simulink model "Fuzzy_Regulator"  (Simulink 7.1)
settings: Solver=ode3  StartTime=0.0  StopTime=30  FixedStep=0.01  RelTol=1e-3
libraries: fuzblock x2, simulink_extras x1, simulink x1
settings Model: Creator=Michal  LastModifiedBy=Michal

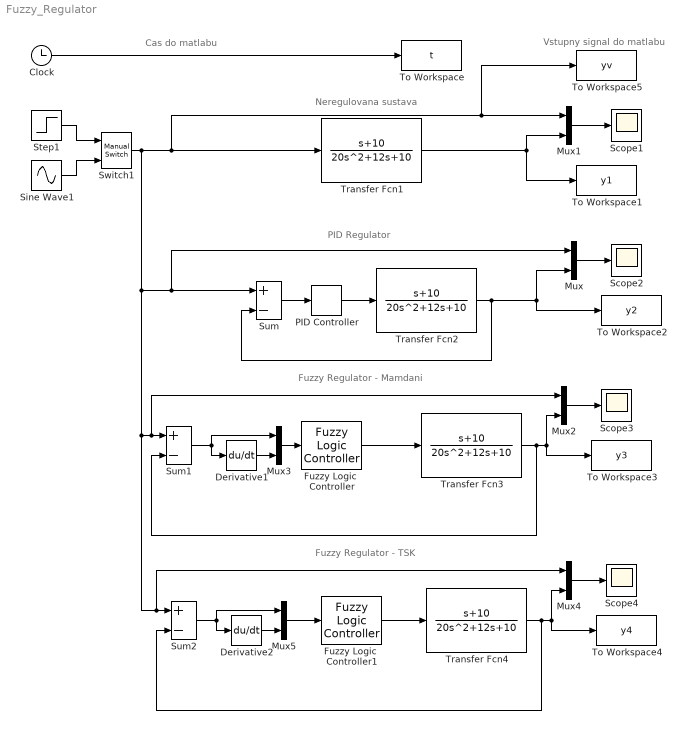
== system Fuzzy_Regulator ==
  note: Cas do matlabu
  note: Neregulovana sustava
  note: PID Regulator
  note: Fuzzy Regulator - Mamdani
  note: Fuzzy Regulator - TSK
  note: Vstupny signal do matlabu
  Clock : Clock
      settings: Decimation=10
  Derivative1 : Derivative
  Derivative2 : Derivative
  Fuzzy Logic  Controller : fuzblock/Fuzzy Logic  Controller  SystemSampleTime=-1  fis='FR_Mamdani.fis'
  Fuzzy Logic  Controller1 : fuzblock/Fuzzy Logic  Controller  SystemSampleTime=-1  fis='FR_TSK.fis'
  Mux{,1..5} (6 alike) : Mux  Inputs=2
  PID Controller : simulink_extras/Additional Linear/PID Controller  SystemSampleTime=-1  P=40  I=2.75  D=20
  Scope{1..4} (4 alike) : Scope
      Scope1 settings: YMin=-4.5e+287  YMax=4.5e+287
      Scope2 settings: YMin=0
      Scope3 settings: YMin=0  SaveName=ScopeData2
      Scope4 settings: TimeRange=20  YMin=-10  YMax=40  SaveName=ScopeData3
  Sine Wave1 : Sin  Bias=10  SampleTime=0
  Step1 : Step  Time=0  After=10  SampleTime=0
  Sum : Sum  Inputs=+|-  OutDataType=sfix(16)  OutScaling=2^0
  Sum1 : Sum  Inputs=+|-  OutDataType=sfix(16)  OutScaling=2^0
  Sum2 : Sum  Inputs=+|-  OutDataType=sfix(16)  OutScaling=2^0
  Switch1 : simulink/Signal Routing/Manual Switch  SystemSampleTime=-1  sw=1  action=0  varsize=off
  To Workspace : ToWorkspace  VariableName=t  SampleTime=-1  SaveFormat=Array
  To Workspace1 : ToWorkspace  VariableName=y1  SampleTime=-1  SaveFormat=Array
  To Workspace2 : ToWorkspace  VariableName=y2  SampleTime=-1  SaveFormat=Array
  To Workspace3 : ToWorkspace  VariableName=y3  SampleTime=-1  SaveFormat=Array
  To Workspace4 : ToWorkspace  VariableName=y4  SampleTime=-1  SaveFormat=Array
  To Workspace5 : ToWorkspace  VariableName=yv  SampleTime=-1  SaveFormat=Array
  Transfer Fcn{1..4} (4 alike) : TransferFcn  Numerator=[1 10]  Denominator=[20 12 10]
  wires:
  Transfer Fcn2/1 -> Sum/2, Mux/2, To Workspace2/1
  PID Controller/1 -> Transfer Fcn2/1
  Sum/1 -> PID Controller/1
  Mux/1 -> Scope2/1
  Mux1/1 -> Scope1/1
  Transfer Fcn1/1 -> Mux1/2, To Workspace1/1
  Transfer Fcn3/1 -> Sum1/2, Mux2/2, To Workspace3/1
  Mux2/1 -> Scope3/1
  Fuzzy Logic  Controller/1 -> Transfer Fcn3/1
  Derivative1/1 -> Mux3/2
  Clock/1 -> To Workspace/1
  Sine Wave1/1 -> Switch1/2
  Step1/1 -> Switch1/1
  Switch1/1 -> Transfer Fcn1/1, Mux1/1, To Workspace5/1, Sum/1, Mux/1, Sum1/1, Mux2/1, Sum2/1, Mux4/1
  Sum1/1 -> Mux3/1, Derivative1/1
  Transfer Fcn4/1 -> Sum2/2, Mux4/2, To Workspace4/1
  Mux4/1 -> Scope4/1
  Fuzzy Logic  Controller1/1 -> Transfer Fcn4/1
  Derivative2/1 -> Mux5/2
  Sum2/1 -> Mux5/1, Derivative2/1
  Mux3/1 -> Fuzzy Logic  Controller/1
  Mux5/1 -> Fuzzy Logic  Controller1/1
